simulink model "SL7_2_8"  (R2019b)
settings: Solver=VariableStepAuto  StartTime=0.0  StopTime=10.0  RelTol=1e-3  EnableMultiTasking=on
settings Model: Creator=Administrator  LastModifiedBy=bhisma
settings DataIOCC: LimitDataPoints=on  ReturnWorkspaceOutputs=off
settings OptimizationCC: LifeSpan=inf
settings DebuggingCC: AllowSymbolicDim=off  SFUnexpectedBacktrackingDiag=warning  SFNoUnconditionalDefaultTransitionDiag=warning  SFExecutionAtInitializationDiag=none  ArithmeticOperatorsInVariantConditions=warning
settings ModelReferenceCC: PropagateSignalLabelsOutOfModel=off
settings SFSimCC: SimUseLocalCustomCode=off  CustomCodeUndefinedFunction=UseInterfaceOnly
settings RTWCC: RTWUseLocalCustomCode=off
settings CodeAppCC: StateflowObjectComments=on
settings GRTTargetCC: TargetLangStandard=C89/C90 (ANSI)
settings ConfigComp: CovMetricSettings=dw  CovHtmlReporting=on  CovSaveCumulativeToWorkspaceVar=on  CovSaveSingleToWorkspaceVar=on  CovExternalEMLEnable=off

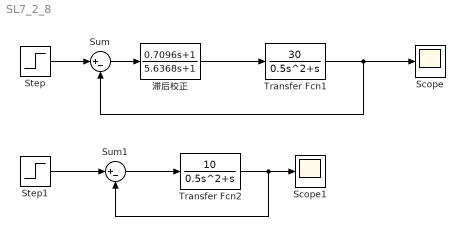
== system SL7_2_8 ==
  Scope : Scope
  Scope1 : Scope
  Step : Step  Time=0  SampleTime=0
  Step1 : Step  Time=0  SampleTime=0
  Sum : Sum  Inputs=|+-
  Sum1 : Sum  Inputs=|+-
  Transfer Fcn1 : TransferFcn  Numerator=[30]  Denominator=[0.5 1 0]
  Transfer Fcn2 : TransferFcn  Numerator=[10]  Denominator=[0.5 1 0]
  滞后校正 : TransferFcn  Numerator=[0.7096 1]  Denominator=[5.6368 1]
  wires:
  滞后校正/1 -> Transfer Fcn1/1
  Sum/1 -> 滞后校正/1
  Step/1 -> Sum/1
  Transfer Fcn1/1 -> Sum/2, Scope/1
  Transfer Fcn2/1 -> Sum1/2, Scope1/1
  Sum1/1 -> Transfer Fcn2/1
  Step1/1 -> Sum1/1
